simulink model "TST_FanCtl_Spd"  (R2016b)
settings: Solver=FixedStepDiscrete  StartTime=0.0  StopTime=simTime  FixedStep=sampleTime  RelTol=1e-3
values from neighbouring files (symbols this model uses):
  testCase = 1    [initTST_FanCtl_Spd_001.m]
libraries: simulink x10, UnitTest_Lib x8
settings Model: Creator=xinchangran  LastModifiedBy=xinchangran
settings DebuggingCC: SignalRangeChecking=error

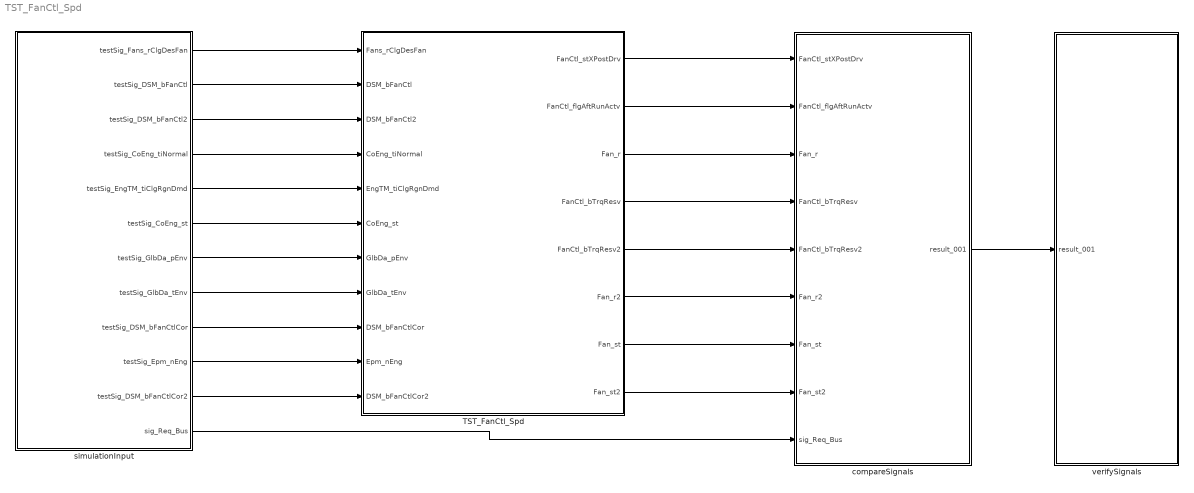
== system TST_FanCtl_Spd ==
  TST_FanCtl_Spd : Subsystem
  compareSignals : Subsystem
  simulationInput : Subsystem
  verifySignals : Subsystem
  wires:
  simulationInput/1(testSig_Fans_rClgDesFan) -> TST_FanCtl_Spd/1(Fans_rClgDesFan)
  simulationInput/2(testSig_DSM_bFanCtl) -> TST_FanCtl_Spd/2(DSM_bFanCtl)
  simulationInput/3(testSig_DSM_bFanCtl2) -> TST_FanCtl_Spd/3(DSM_bFanCtl2)
  simulationInput/4(testSig_CoEng_tiNormal) -> TST_FanCtl_Spd/4(CoEng_tiNormal)
  simulationInput/5(testSig_EngTM_tiClgRgnDmd) -> TST_FanCtl_Spd/5(EngTM_tiClgRgnDmd)
  simulationInput/6(testSig_CoEng_st) -> TST_FanCtl_Spd/6(CoEng_st)
  simulationInput/7(testSig_GlbDa_pEnv) -> TST_FanCtl_Spd/7(GlbDa_pEnv)
  simulationInput/8(testSig_GlbDa_tEnv) -> TST_FanCtl_Spd/8(GlbDa_tEnv)
  simulationInput/9(testSig_DSM_bFanCtlCor) -> TST_FanCtl_Spd/9(DSM_bFanCtlCor)
  simulationInput/10(testSig_Epm_nEng) -> TST_FanCtl_Spd/10(Epm_nEng)
  simulationInput/11(testSig_DSM_bFanCtlCor2) -> TST_FanCtl_Spd/11(DSM_bFanCtlCor2)
  TST_FanCtl_Spd/1(FanCtl_stXPostDrv) -> compareSignals/1(FanCtl_stXPostDrv)
  TST_FanCtl_Spd/2(FanCtl_flgAftRunActv) -> compareSignals/2(FanCtl_flgAftRunActv)
  TST_FanCtl_Spd/3(Fan_r) -> compareSignals/3(Fan_r)
  TST_FanCtl_Spd/4(FanCtl_bTrqResv) -> compareSignals/4(FanCtl_bTrqResv)
  TST_FanCtl_Spd/5(FanCtl_bTrqResv2) -> compareSignals/5(FanCtl_bTrqResv2)
  TST_FanCtl_Spd/6(Fan_r2) -> compareSignals/6(Fan_r2)
  TST_FanCtl_Spd/7(Fan_st) -> compareSignals/7(Fan_st)
  TST_FanCtl_Spd/8(Fan_st2) -> compareSignals/8(Fan_st2)
  simulationInput/12(sig_Req_Bus) -> compareSignals/9(sig_Req_Bus)
  compareSignals/1(result_001) -> verifySignals/1(result_001)

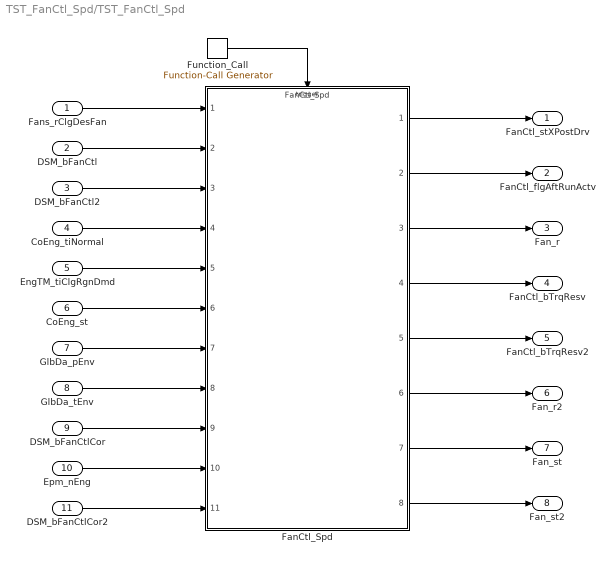
== system TST_FanCtl_Spd/TST_FanCtl_Spd ==
  Fans_rClgDesFan : Inport
  DSM_bFanCtl : Inport  Port=2
  DSM_bFanCtl2 : Inport  Port=3
  CoEng_tiNormal : Inport  Port=4
  EngTM_tiClgRgnDmd : Inport  Port=5
  CoEng_st : Inport  Port=6
  GlbDa_pEnv : Inport  Port=7
  GlbDa_tEnv : Inport  Port=8
  DSM_bFanCtlCor : Inport  Port=9
  Epm_nEng : Inport  Port=10
  DSM_bFanCtlCor2 : Inport  Port=11
  FanCtl_Spd : ModelReference  ModelNameDialog=FanCtl_Spd  SimulationMode=Normal  ModelReferenceVersion=1.190  TriggerPortName=function  TriggerPortTriggerType=function-call  TriggerPortStatesWhenEnabling=held
  Function_Call : simulink/Ports & Subsystems/Function-Call Generator  sample_time=sampleTime  numberOfIterations=1
  FanCtl_stXPostDrv : Outport
  FanCtl_flgAftRunActv : Outport  Port=2
  Fan_r : Outport  Port=3
  FanCtl_bTrqResv : Outport  Port=4
  FanCtl_bTrqResv2 : Outport  Port=5
  Fan_r2 : Outport  Port=6
  Fan_st : Outport  Port=7
  Fan_st2 : Outport  Port=8
  wires:
  Function_Call/1 -> FanCtl_Spd/Trigger
  Fans_rClgDesFan/1 -> FanCtl_Spd/1
  DSM_bFanCtl/1 -> FanCtl_Spd/2
  DSM_bFanCtl2/1 -> FanCtl_Spd/3
  CoEng_tiNormal/1 -> FanCtl_Spd/4
  EngTM_tiClgRgnDmd/1 -> FanCtl_Spd/5
  CoEng_st/1 -> FanCtl_Spd/6
  GlbDa_pEnv/1 -> FanCtl_Spd/7
  GlbDa_tEnv/1 -> FanCtl_Spd/8
  DSM_bFanCtlCor/1 -> FanCtl_Spd/9
  Epm_nEng/1 -> FanCtl_Spd/10
  DSM_bFanCtlCor2/1 -> FanCtl_Spd/11
  FanCtl_Spd/1 -> FanCtl_stXPostDrv/1
  FanCtl_Spd/2 -> FanCtl_flgAftRunActv/1
  FanCtl_Spd/3 -> Fan_r/1
  FanCtl_Spd/4 -> FanCtl_bTrqResv/1
  FanCtl_Spd/5 -> FanCtl_bTrqResv2/1
  FanCtl_Spd/6 -> Fan_r2/1
  FanCtl_Spd/7 -> Fan_st/1
  FanCtl_Spd/8 -> Fan_st2/1

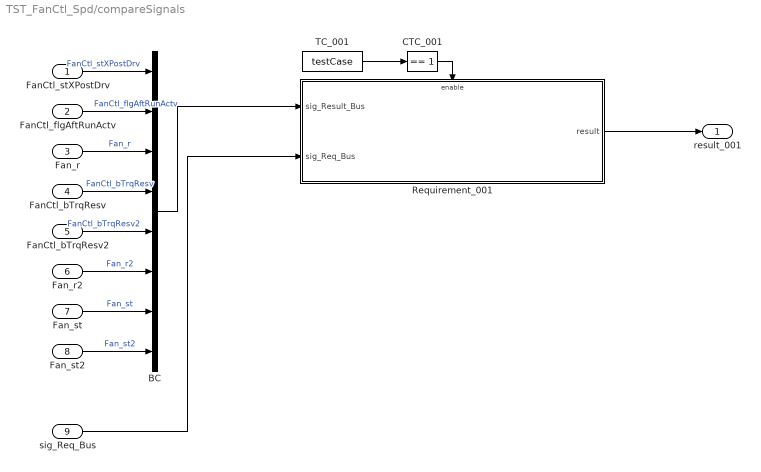
== system TST_FanCtl_Spd/compareSignals ==
  FanCtl_stXPostDrv : Inport
  FanCtl_flgAftRunActv : Inport  Port=2
  Fan_r : Inport  Port=3
  FanCtl_bTrqResv : Inport  Port=4
  FanCtl_bTrqResv2 : Inport  Port=5
  Fan_r2 : Inport  Port=6
  Fan_st : Inport  Port=7
  Fan_st2 : Inport  Port=8
  sig_Req_Bus : Inport  Port=9
  BC : BusCreator  Inputs=8
  CTC_001 : simulink/Logic and Bit Operations/Compare To Constant  relop===  const=1  OutDataTypeStr=boolean
  Requirement_001 : Subsystem
  TC_001 : Constant  Value=testCase
  result_001 : Outport
  wires:
  FanCtl_stXPostDrv/1 -> BC/1  "FanCtl_stXPostDrv"
  FanCtl_flgAftRunActv/1 -> BC/2  "FanCtl_flgAftRunActv"
  Fan_r/1 -> BC/3  "Fan_r"
  FanCtl_bTrqResv/1 -> BC/4  "FanCtl_bTrqResv"
  FanCtl_bTrqResv2/1 -> BC/5  "FanCtl_bTrqResv2"
  Fan_r2/1 -> BC/6  "Fan_r2"
  Fan_st/1 -> BC/7  "Fan_st"
  Fan_st2/1 -> BC/8  "Fan_st2"
  TC_001/1 -> CTC_001/1
  CTC_001/1 -> Requirement_001/Enable
  sig_Req_Bus/1 -> Requirement_001/2(sig_Req_Bus)
  BC/1 -> Requirement_001/1(sig_Result_Bus)
  Requirement_001/1(result) -> result_001/1

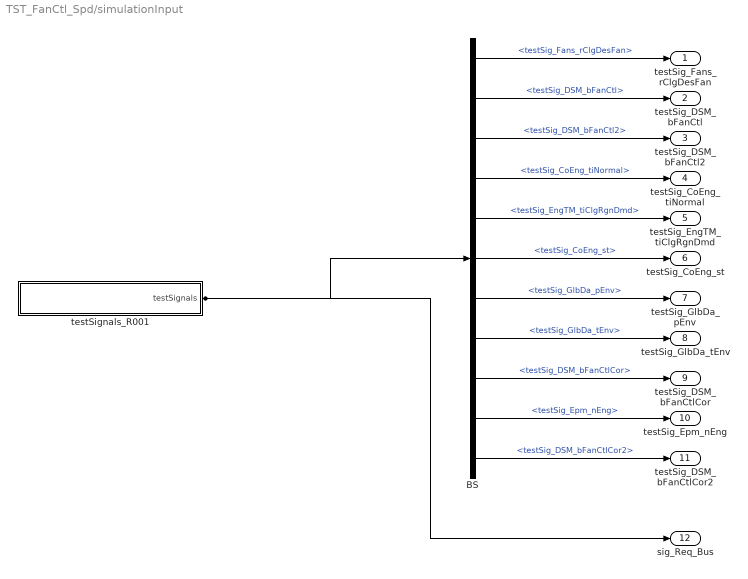
== system TST_FanCtl_Spd/simulationInput ==
  BS : BusSelector  OutputSignals=testSig_Fans_rClgDesFan,testSig_DSM_bFanCtl,testSig_DSM_bFanCtl2,testSig_CoEng_tiNormal,testSig_EngTM_tiClgRgnDmd,testSig_CoEng_st,testSig_GlbDa_pEnv,testSig_GlbDa_tEnv,testSig_DSM_bFanCtlCor,testSig_Epm_nEng,testSig_DSM_bFanCtlCor2
  testSignals_R001 : Subsystem
  testSig_Fans_rClgDesFan : Outport
  testSig_DSM_bFanCtl : Outport  Port=2
  testSig_DSM_bFanCtl2 : Outport  Port=3
  testSig_CoEng_tiNormal : Outport  Port=4
  testSig_EngTM_tiClgRgnDmd : Outport  Port=5
  testSig_CoEng_st : Outport  Port=6
  testSig_GlbDa_pEnv : Outport  Port=7
  testSig_GlbDa_tEnv : Outport  Port=8
  testSig_DSM_bFanCtlCor : Outport  Port=9
  testSig_Epm_nEng : Outport  Port=10
  testSig_DSM_bFanCtlCor2 : Outport  Port=11
  sig_Req_Bus : Outport  Port=12
  wires:
  BS/1 -> testSig_Fans_rClgDesFan/1  "<testSig_Fans_rClgDesFan>"
  BS/2 -> testSig_DSM_bFanCtl/1  "<testSig_DSM_bFanCtl>"
  BS/3 -> testSig_DSM_bFanCtl2/1  "<testSig_DSM_bFanCtl2>"
  BS/4 -> testSig_CoEng_tiNormal/1  "<testSig_CoEng_tiNormal>"
  BS/5 -> testSig_EngTM_tiClgRgnDmd/1  "<testSig_EngTM_tiClgRgnDmd>"
  BS/6 -> testSig_CoEng_st/1  "<testSig_CoEng_st>"
  BS/7 -> testSig_GlbDa_pEnv/1  "<testSig_GlbDa_pEnv>"
  BS/8 -> testSig_GlbDa_tEnv/1  "<testSig_GlbDa_tEnv>"
  BS/9 -> testSig_DSM_bFanCtlCor/1  "<testSig_DSM_bFanCtlCor>"
  BS/10 -> testSig_Epm_nEng/1  "<testSig_Epm_nEng>"
  BS/11 -> testSig_DSM_bFanCtlCor2/1  "<testSig_DSM_bFanCtlCor2>"
  testSignals_R001/1(testSignals) -> BS/1, sig_Req_Bus/1

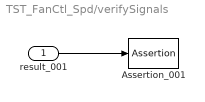
== system TST_FanCtl_Spd/verifySignals ==
  result_001 : Inport
  Assertion_001 : Assertion  Enabled=off
  wires:
  result_001/1 -> Assertion_001/1

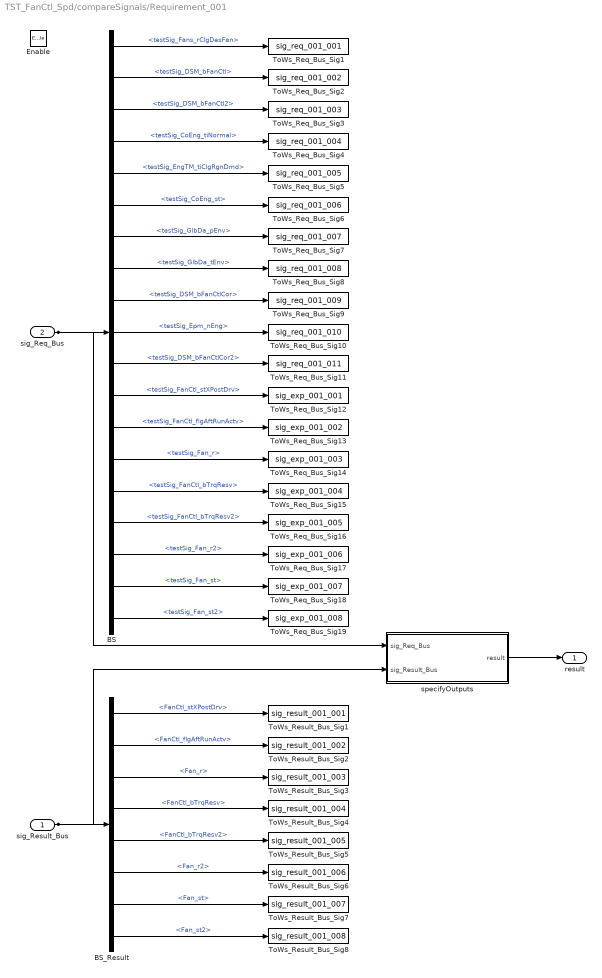
== system TST_FanCtl_Spd/compareSignals/Requirement_001 ==
  sig_Result_Bus : Inport
  sig_Req_Bus : Inport  Port=2
  Enable : EnablePort
  BS : BusSelector  OutputSignals=testSig_Fans_rClgDesFan,testSig_DSM_bFanCtl,testSig_DSM_bFanCtl2,testSig_CoEng_tiNormal,testSig_EngTM_tiClgRgnDmd,testSig_CoEng_st,testSig_GlbDa_pEnv,testSig_GlbDa_tEnv,testSig_DSM_bFanCtlCor,testSig_Epm_nEng,testSig_DSM_bFanCtlCor2,testSig_FanCtl_stXPostDrv,testSig_FanCtl_flgAftRunActv,testSig_Fan_r,testSig_FanCtl_bTrqResv,testSig_FanCtl_bTrqResv2,testSig_Fan_r2,testSig_Fan_st,testSig_Fan_st2
  BS_Result : BusSelector  OutputSignals=FanCtl_stXPostDrv,FanCtl_flgAftRunActv,Fan_r,FanCtl_bTrqResv,FanCtl_bTrqResv2,Fan_r2,Fan_st,Fan_st2
  ToWs_Req_Bus_Sig1 : ToWorkspace  VariableName=sig_req_001_001  SaveFormat=Structure With Time
  ToWs_Req_Bus_Sig10 : ToWorkspace  VariableName=sig_req_001_010  SaveFormat=Structure With Time
  ToWs_Req_Bus_Sig11 : ToWorkspace  VariableName=sig_req_001_011  SaveFormat=Structure With Time
  ToWs_Req_Bus_Sig12 : ToWorkspace  VariableName=sig_exp_001_001  SaveFormat=Structure With Time
  ToWs_Req_Bus_Sig13 : ToWorkspace  VariableName=sig_exp_001_002  SaveFormat=Structure With Time
  ToWs_Req_Bus_Sig14 : ToWorkspace  VariableName=sig_exp_001_003  SaveFormat=Structure With Time
  ToWs_Req_Bus_Sig15 : ToWorkspace  VariableName=sig_exp_001_004  SaveFormat=Structure With Time
  ToWs_Req_Bus_Sig16 : ToWorkspace  VariableName=sig_exp_001_005  SaveFormat=Structure With Time
  ToWs_Req_Bus_Sig17 : ToWorkspace  VariableName=sig_exp_001_006  SaveFormat=Structure With Time
  ToWs_Req_Bus_Sig18 : ToWorkspace  VariableName=sig_exp_001_007  SaveFormat=Structure With Time
  ToWs_Req_Bus_Sig19 : ToWorkspace  VariableName=sig_exp_001_008  SaveFormat=Structure With Time
  ToWs_Req_Bus_Sig2 : ToWorkspace  VariableName=sig_req_001_002  SaveFormat=Structure With Time
  ToWs_Req_Bus_Sig3 : ToWorkspace  VariableName=sig_req_001_003  SaveFormat=Structure With Time
  ToWs_Req_Bus_Sig4 : ToWorkspace  VariableName=sig_req_001_004  SaveFormat=Structure With Time
  ToWs_Req_Bus_Sig5 : ToWorkspace  VariableName=sig_req_001_005  SaveFormat=Structure With Time
  ToWs_Req_Bus_Sig6 : ToWorkspace  VariableName=sig_req_001_006  SaveFormat=Structure With Time
  ToWs_Req_Bus_Sig7 : ToWorkspace  VariableName=sig_req_001_007  SaveFormat=Structure With Time
  ToWs_Req_Bus_Sig8 : ToWorkspace  VariableName=sig_req_001_008  SaveFormat=Structure With Time
  ToWs_Req_Bus_Sig9 : ToWorkspace  VariableName=sig_req_001_009  SaveFormat=Structure With Time
  ToWs_Result_Bus_Sig1 : ToWorkspace  VariableName=sig_result_001_001  SaveFormat=Structure With Time
  ToWs_Result_Bus_Sig2 : ToWorkspace  VariableName=sig_result_001_002  SaveFormat=Structure With Time
  ToWs_Result_Bus_Sig3 : ToWorkspace  VariableName=sig_result_001_003  SaveFormat=Structure With Time
  ToWs_Result_Bus_Sig4 : ToWorkspace  VariableName=sig_result_001_004  SaveFormat=Structure With Time
  ToWs_Result_Bus_Sig5 : ToWorkspace  VariableName=sig_result_001_005  SaveFormat=Structure With Time
  ToWs_Result_Bus_Sig6 : ToWorkspace  VariableName=sig_result_001_006  SaveFormat=Structure With Time
  ToWs_Result_Bus_Sig7 : ToWorkspace  VariableName=sig_result_001_007  SaveFormat=Structure With Time
  ToWs_Result_Bus_Sig8 : ToWorkspace  VariableName=sig_result_001_008  SaveFormat=Structure With Time
  specifyOutputs : Subsystem
  result : Outport
  wires:
  sig_Req_Bus/1 -> BS/1, specifyOutputs/1(sig_Req_Bus)
  BS/1 -> ToWs_Req_Bus_Sig1/1  "<testSig_Fans_rClgDesFan>"
  BS/2 -> ToWs_Req_Bus_Sig2/1  "<testSig_DSM_bFanCtl>"
  BS/3 -> ToWs_Req_Bus_Sig3/1  "<testSig_DSM_bFanCtl2>"
  BS/4 -> ToWs_Req_Bus_Sig4/1  "<testSig_CoEng_tiNormal>"
  BS/5 -> ToWs_Req_Bus_Sig5/1  "<testSig_EngTM_tiClgRgnDmd>"
  BS/6 -> ToWs_Req_Bus_Sig6/1  "<testSig_CoEng_st>"
  BS/7 -> ToWs_Req_Bus_Sig7/1  "<testSig_GlbDa_pEnv>"
  BS/8 -> ToWs_Req_Bus_Sig8/1  "<testSig_GlbDa_tEnv>"
  BS/9 -> ToWs_Req_Bus_Sig9/1  "<testSig_DSM_bFanCtlCor>"
  BS/10 -> ToWs_Req_Bus_Sig10/1  "<testSig_Epm_nEng>"
  BS/11 -> ToWs_Req_Bus_Sig11/1  "<testSig_DSM_bFanCtlCor2>"
  BS/12 -> ToWs_Req_Bus_Sig12/1  "<testSig_FanCtl_stXPostDrv>"
  BS/13 -> ToWs_Req_Bus_Sig13/1  "<testSig_FanCtl_flgAftRunActv>"
  BS/14 -> ToWs_Req_Bus_Sig14/1  "<testSig_Fan_r>"
  BS/15 -> ToWs_Req_Bus_Sig15/1  "<testSig_FanCtl_bTrqResv>"
  BS/16 -> ToWs_Req_Bus_Sig16/1  "<testSig_FanCtl_bTrqResv2>"
  BS/17 -> ToWs_Req_Bus_Sig17/1  "<testSig_Fan_r2>"
  BS/18 -> ToWs_Req_Bus_Sig18/1  "<testSig_Fan_st>"
  BS/19 -> ToWs_Req_Bus_Sig19/1  "<testSig_Fan_st2>"
  sig_Result_Bus/1 -> BS_Result/1, specifyOutputs/2(sig_Result_Bus)
  BS_Result/1 -> ToWs_Result_Bus_Sig1/1  "<FanCtl_stXPostDrv>"
  BS_Result/2 -> ToWs_Result_Bus_Sig2/1  "<FanCtl_flgAftRunActv>"
  BS_Result/3 -> ToWs_Result_Bus_Sig3/1  "<Fan_r>"
  BS_Result/4 -> ToWs_Result_Bus_Sig4/1  "<FanCtl_bTrqResv>"
  BS_Result/5 -> ToWs_Result_Bus_Sig5/1  "<FanCtl_bTrqResv2>"
  BS_Result/6 -> ToWs_Result_Bus_Sig6/1  "<Fan_r2>"
  BS_Result/7 -> ToWs_Result_Bus_Sig7/1  "<Fan_st>"
  BS_Result/8 -> ToWs_Result_Bus_Sig8/1  "<Fan_st2>"
  specifyOutputs/1(result) -> result/1

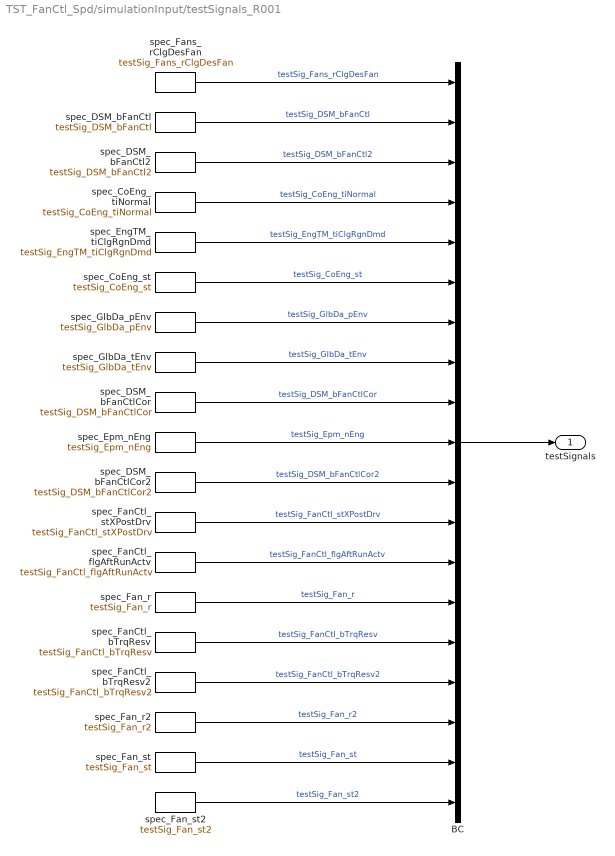
== system TST_FanCtl_Spd/simulationInput/testSignals_R001 ==
  BC : BusCreator  Inputs=19
  spec_CoEng_st : FromWorkspace  VariableName=testSig_CoEng_st  Interpolate=off  OutputAfterFinalValue=Holding final value
  spec_CoEng_tiNormal : FromWorkspace  VariableName=testSig_CoEng_tiNormal  Interpolate=off  OutputAfterFinalValue=Holding final value
  spec_DSM_bFanCtl : FromWorkspace  VariableName=testSig_DSM_bFanCtl  Interpolate=off  OutputAfterFinalValue=Holding final value
  spec_DSM_bFanCtl2 : FromWorkspace  VariableName=testSig_DSM_bFanCtl2  Interpolate=off  OutputAfterFinalValue=Holding final value
  spec_DSM_bFanCtlCor : FromWorkspace  VariableName=testSig_DSM_bFanCtlCor  Interpolate=off  OutputAfterFinalValue=Holding final value
  spec_DSM_bFanCtlCor2 : FromWorkspace  VariableName=testSig_DSM_bFanCtlCor2  Interpolate=off  OutputAfterFinalValue=Holding final value
  spec_EngTM_tiClgRgnDmd : FromWorkspace  VariableName=testSig_EngTM_tiClgRgnDmd  Interpolate=off  OutputAfterFinalValue=Holding final value
  spec_Epm_nEng : FromWorkspace  VariableName=testSig_Epm_nEng  Interpolate=off  OutputAfterFinalValue=Holding final value
  spec_FanCtl_bTrqResv : FromWorkspace  VariableName=testSig_FanCtl_bTrqResv  Interpolate=off  OutputAfterFinalValue=Holding final value
  spec_FanCtl_bTrqResv2 : FromWorkspace  VariableName=testSig_FanCtl_bTrqResv2  Interpolate=off  OutputAfterFinalValue=Holding final value
  spec_FanCtl_flgAftRunActv : FromWorkspace  VariableName=testSig_FanCtl_flgAftRunActv  Interpolate=off  OutputAfterFinalValue=Holding final value
  spec_FanCtl_stXPostDrv : FromWorkspace  VariableName=testSig_FanCtl_stXPostDrv  Interpolate=off  OutputAfterFinalValue=Holding final value
  spec_Fan_r : FromWorkspace  VariableName=testSig_Fan_r  Interpolate=off  OutputAfterFinalValue=Holding final value
  spec_Fan_r2 : FromWorkspace  VariableName=testSig_Fan_r2  Interpolate=off  OutputAfterFinalValue=Holding final value
  spec_Fan_st : FromWorkspace  VariableName=testSig_Fan_st  Interpolate=off  OutputAfterFinalValue=Holding final value
  spec_Fan_st2 : FromWorkspace  VariableName=testSig_Fan_st2  Interpolate=off  OutputAfterFinalValue=Holding final value
  spec_Fans_rClgDesFan : FromWorkspace  VariableName=testSig_Fans_rClgDesFan  Interpolate=off  OutputAfterFinalValue=Holding final value
  spec_GlbDa_pEnv : FromWorkspace  VariableName=testSig_GlbDa_pEnv  Interpolate=off  OutputAfterFinalValue=Holding final value
  spec_GlbDa_tEnv : FromWorkspace  VariableName=testSig_GlbDa_tEnv  Interpolate=off  OutputAfterFinalValue=Holding final value
  testSignals : Outport
  wires:
  BC/1 -> testSignals/1
  spec_Fans_rClgDesFan/1 -> BC/1  "testSig_Fans_rClgDesFan"
  spec_DSM_bFanCtl/1 -> BC/2  "testSig_DSM_bFanCtl"
  spec_DSM_bFanCtl2/1 -> BC/3  "testSig_DSM_bFanCtl2"
  spec_CoEng_tiNormal/1 -> BC/4  "testSig_CoEng_tiNormal"
  spec_EngTM_tiClgRgnDmd/1 -> BC/5  "testSig_EngTM_tiClgRgnDmd"
  spec_CoEng_st/1 -> BC/6  "testSig_CoEng_st"
  spec_GlbDa_pEnv/1 -> BC/7  "testSig_GlbDa_pEnv"
  spec_GlbDa_tEnv/1 -> BC/8  "testSig_GlbDa_tEnv"
  spec_DSM_bFanCtlCor/1 -> BC/9  "testSig_DSM_bFanCtlCor"
  spec_Epm_nEng/1 -> BC/10  "testSig_Epm_nEng"
  spec_DSM_bFanCtlCor2/1 -> BC/11  "testSig_DSM_bFanCtlCor2"
  spec_FanCtl_stXPostDrv/1 -> BC/12  "testSig_FanCtl_stXPostDrv"
  spec_FanCtl_flgAftRunActv/1 -> BC/13  "testSig_FanCtl_flgAftRunActv"
  spec_Fan_r/1 -> BC/14  "testSig_Fan_r"
  spec_FanCtl_bTrqResv/1 -> BC/15  "testSig_FanCtl_bTrqResv"
  spec_FanCtl_bTrqResv2/1 -> BC/16  "testSig_FanCtl_bTrqResv2"
  spec_Fan_r2/1 -> BC/17  "testSig_Fan_r2"
  spec_Fan_st/1 -> BC/18  "testSig_Fan_st"
  spec_Fan_st2/1 -> BC/19  "testSig_Fan_st2"

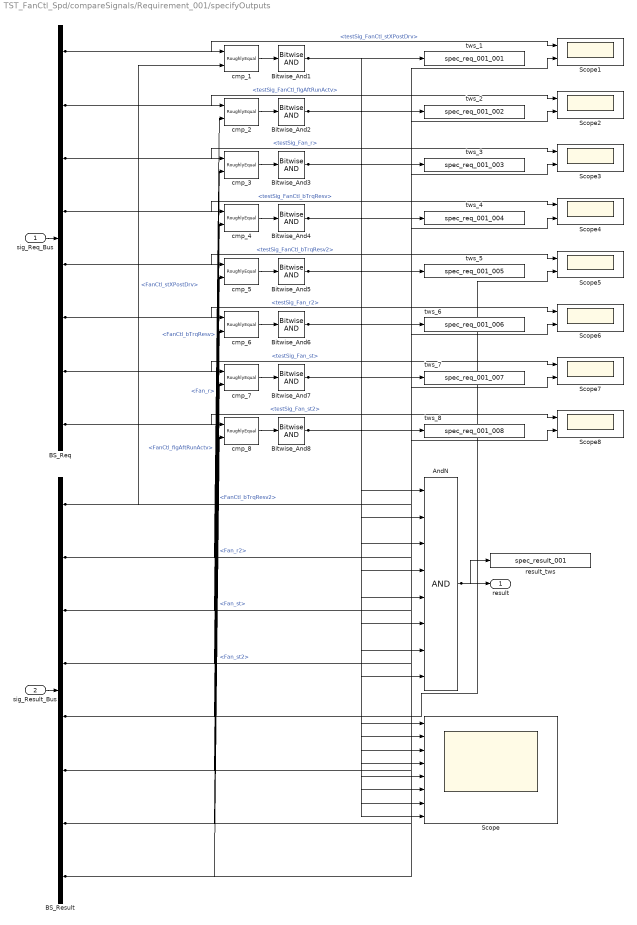
== system TST_FanCtl_Spd/compareSignals/Requirement_001/specifyOutputs ==
  sig_Req_Bus : Inport
  sig_Result_Bus : Inport  Port=2
  AndN : Logic  Inputs=8
  BS_Req : BusSelector  OutputSignals=testSig_FanCtl_stXPostDrv,testSig_FanCtl_flgAftRunActv,testSig_Fan_r,testSig_FanCtl_bTrqResv,testSig_FanCtl_bTrqResv2,testSig_Fan_r2,testSig_Fan_st,testSig_Fan_st2
  BS_Result : BusSelector  OutputSignals=FanCtl_stXPostDrv,FanCtl_flgAftRunActv,Fan_r,FanCtl_bTrqResv,FanCtl_bTrqResv2,Fan_r2,Fan_st,Fan_st2
  Bitwise_And{1..8} (8 alike) : simulink/Logic and Bit Operations/Bitwise Operator  logicop=AND  UseBitMask=off  BitMask=bin2dec('11011001')  BitMaskRealWorld=Stored Integer
  Scope : Scope  NumInputPorts=8
  Scope{1..8} (8 alike) : Scope  NumInputPorts=2
  cmp_{1..8} (8 alike) : UnitTest_Lib/RoughlyEqual  slope=0.1
  result_tws : ToWorkspace  VariableName=spec_result_001
  tws_1 : ToWorkspace  VariableName=spec_req_001_001
  tws_2 : ToWorkspace  VariableName=spec_req_001_002
  tws_3 : ToWorkspace  VariableName=spec_req_001_003
  tws_4 : ToWorkspace  VariableName=spec_req_001_004
  tws_5 : ToWorkspace  VariableName=spec_req_001_005
  tws_6 : ToWorkspace  VariableName=spec_req_001_006
  tws_7 : ToWorkspace  VariableName=spec_req_001_007
  tws_8 : ToWorkspace  VariableName=spec_req_001_008
  result : Outport
  wires:
  sig_Req_Bus/1 -> BS_Req/1
  sig_Result_Bus/1 -> BS_Result/1
  AndN/1 -> result/1, result_tws/1
  BS_Req/1 -> cmp_1/1, Scope1/1  "<testSig_FanCtl_stXPostDrv>"
  BS_Result/1 -> cmp_1/2, Scope1/2  "<FanCtl_stXPostDrv>"
  cmp_1/1 -> Bitwise_And1/1
  Bitwise_And1/1 -> tws_1/1, AndN/1, Scope/1
  BS_Req/2 -> cmp_2/1, Scope2/1  "<testSig_FanCtl_flgAftRunActv>"
  BS_Result/2 -> cmp_2/2, Scope2/2  "<FanCtl_flgAftRunActv>"
  cmp_2/1 -> Bitwise_And2/1
  Bitwise_And2/1 -> tws_2/1, AndN/2, Scope/2
  BS_Req/3 -> cmp_3/1, Scope3/1  "<testSig_Fan_r>"
  BS_Result/3 -> cmp_3/2, Scope3/2  "<Fan_r>"
  cmp_3/1 -> Bitwise_And3/1
  Bitwise_And3/1 -> tws_3/1, AndN/3, Scope/3
  BS_Req/4 -> cmp_4/1, Scope4/1  "<testSig_FanCtl_bTrqResv>"
  BS_Result/4 -> cmp_4/2, Scope4/2  "<FanCtl_bTrqResv>"
  cmp_4/1 -> Bitwise_And4/1
  Bitwise_And4/1 -> tws_4/1, AndN/4, Scope/4
  BS_Req/5 -> cmp_5/1, Scope5/1  "<testSig_FanCtl_bTrqResv2>"
  BS_Result/5 -> cmp_5/2, Scope5/2  "<FanCtl_bTrqResv2>"
  cmp_5/1 -> Bitwise_And5/1
  Bitwise_And5/1 -> tws_5/1, AndN/5, Scope/5
  BS_Req/6 -> cmp_6/1, Scope6/1  "<testSig_Fan_r2>"
  BS_Result/6 -> cmp_6/2, Scope6/2  "<Fan_r2>"
  cmp_6/1 -> Bitwise_And6/1
  Bitwise_And6/1 -> tws_6/1, AndN/6, Scope/6
  BS_Req/7 -> cmp_7/1, Scope7/1  "<testSig_Fan_st>"
  BS_Result/7 -> cmp_7/2, Scope7/2  "<Fan_st>"
  cmp_7/1 -> Bitwise_And7/1
  Bitwise_And7/1 -> tws_7/1, AndN/7, Scope/7
  BS_Req/8 -> cmp_8/1, Scope8/1  "<testSig_Fan_st2>"
  BS_Result/8 -> cmp_8/2, Scope8/2  "<Fan_st2>"
  cmp_8/1 -> Bitwise_And8/1
  Bitwise_And8/1 -> tws_8/1, AndN/8, Scope/8
